simulink model "TrajectoryGeneration"  (R2023a)
settings: Solver=VariableStepAuto  StartTime=0.0  StopTime=10  RelTol=1e-3
libraries: dspnetwork x2
settings Model: Creator=skala  LastModifiedBy=jeric
settings ModelReferenceCC: EnableRefExpFcnMdlSchedulingChecks=on

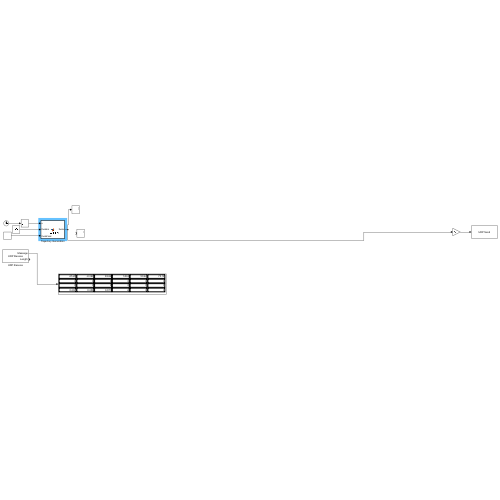
[thumbnail: Simulink's stored preview of the top-level diagram]
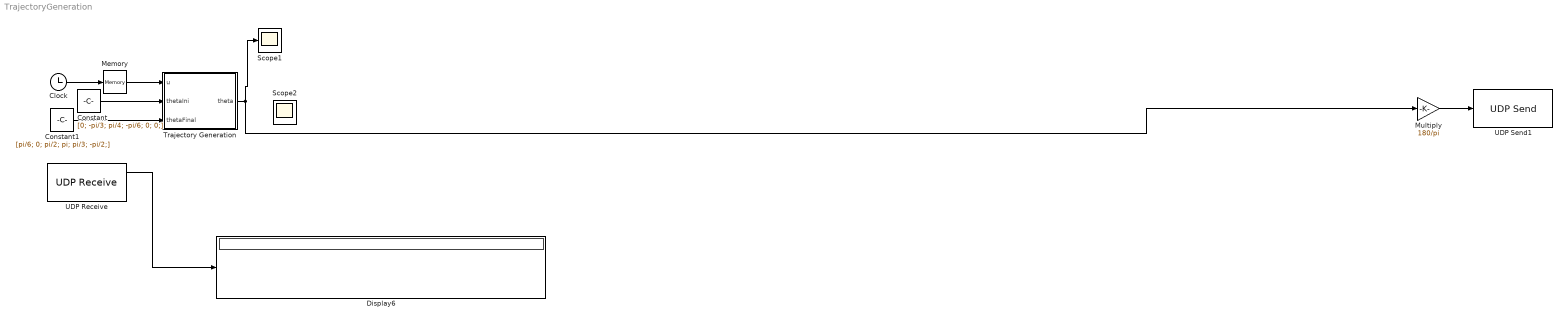
== system TrajectoryGeneration ==
  Clock : Clock
  Constant : Constant  Value=[0; -pi/3; pi/4; -pi/6; 0; 0;]
  Constant1 : Constant  Value=[pi/6; 0; pi/2; pi; pi/3; -pi/2;]
  Display6 : Display
  Memory : Memory  InheritSampleTime=on
  Multiply : Gain  Gain=180/pi
  Scope1 : Scope
  Scope2 : Scope
  Trajectory Generation : MATLAB Function  TreatAsAtomicUnit=on
  UDP Receive : dspnetwork/UDP Receive  localURL='0.0.0.0'  localPort=28008  remoteURL='127.0.0.1'  remotePort=-1  recvBufferSize=2500  dims=24  signalDatatype=double  isComplex=off  isVarSize=off  showBlockingTime=off  blockingTime=0  sampletime=.0001  blockPlatform=[]
      settings: LibrarySourceBlock=dspsrcs4/UDP Receive
  UDP Send1 : dspnetwork/UDP Send  remoteURL='127.0.0.1'  remotePort=28007  localURL='0.0.0.0'  localPortSource=Automatically determine  localPort=-1  sendBufferSize=8192  sampletime=-1  blockPlatform=[]  separateLengthPort=0
      settings: LibrarySourceBlock=dspsnks4/UDP Send
  wires:
  Clock/1 -> Memory/1
  Trajectory Generation/1(theta) -> Multiply/1, Scope1/1
  Multiply/1 -> UDP Send1/1
  Memory/1 -> Trajectory Generation/1(u)
  UDP Receive/1 -> Display6/1
  Constant/1 -> Trajectory Generation/2(thetaIni)
  Constant1/1 -> Trajectory Generation/3(thetaFinal)

== matlab function TrajectoryGeneration/Trajectory Generation ==
  data: u input; thetaIni input; theta output; thetaFinal input
function theta  = TRAJGEN(u, thetaIni, thetaFinal)

tf = 10;

matrix = [tf^3, tf^2; 3 * tf^2, 2 * tf;];

theta = zeros(6, 1);

for i = 1 : 6
    vector = matrix \ [thetaFinal(i) - thetaIni(i); 0];
    theta(i) = vector(1) * u ^ 3 + vector(2) * u ^ 2 + thetaIni(i);
end
